simulink model "finger_model_based_control_v2"  (Simulink 6.6)
settings: Solver=ode3  StartTime=0.0  StopTime=5  FixedStep=0.01  RelTol=1e-3
undefined symbols (not defined in the file or in its folder): get
libraries: simulink x5, dspinverses x1, dspsnks4 x1
settings Model: Creator=Jadav Das  LastModifiedBy=Jadav Das
settings OptimizationCC: InlineInvariantSignals=on
settings DebuggingCC: SignalResolutionControl=TryResolveAllWithWarning  MultiTaskDSMMsg=warning  MultiTaskCondExecSysMsg=none  StrictBusMsg=None
settings RTWCC: IncludeERTFirstTime=on

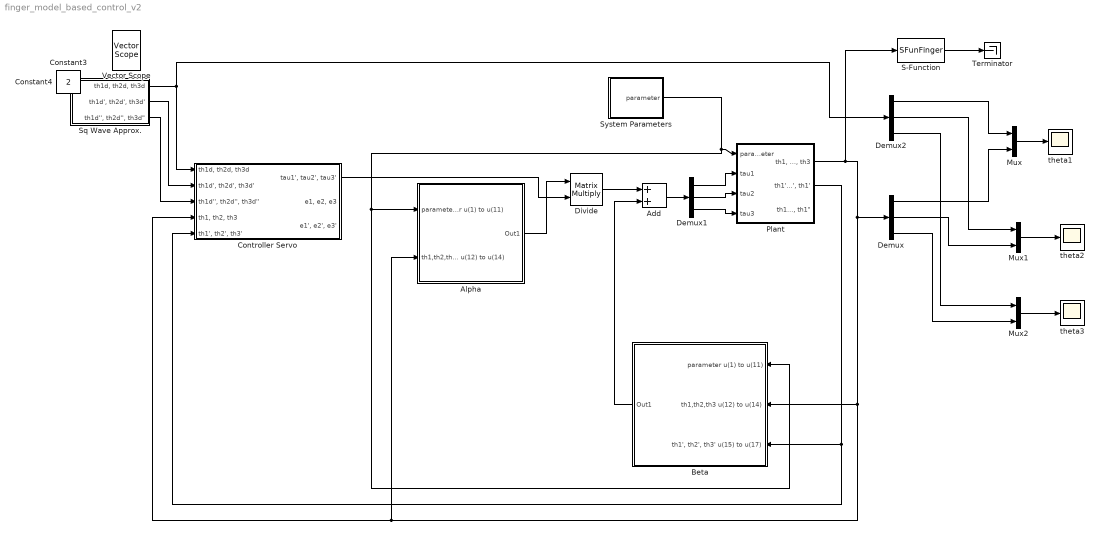
== system finger_model_based_control_v2 ==
  Add : Sum  OutScaling=2^-10
  Alpha : Subsystem
  Beta : Subsystem  Orientation=left
  Controller Servo : Subsystem
  Demux : Demux  Outputs=3
  Demux1 : Demux  Outputs=3
  Demux2 : Demux  Outputs=3
  Divide : Product  Inputs=**  Multiplication=Matrix(*)  OutScaling=2^-10
  Mux : Mux  Inputs=2
  Mux1 : Mux  Inputs=2
  Mux2 : Mux  Inputs=2
  Plant : Subsystem
  S-Function : S-Function  FunctionName=SFunFinger
  Sq Wave Approx. : Subsystem
  System Parameters : Subsystem
  Terminator : Terminator
  theta1 : Scope
      settings: TimeRange=40
  theta2 : Scope
      settings: TimeRange=40  SaveName=ScopeData2
  theta3 : Scope
      settings: TimeRange=40  SaveName=ScopeData3
  Constant3 : Constant  IOType=siggen  Value=0.5
  Constant4 : Constant  IOType=siggen  Value=2
  Vector Scope : dspsnks4/Vector Scope  IOType=viewer  DialogController=dspdialog.VectorScope  DialogControllerArgs=DataTag0  ScopeProperties=on  Domain=Time  HorizSpan=1  DisplayProperties=off  AxisGrid=off  Memory=off  FrameNumber=off  AxisLegend=off  AxisZoom=off  OpenScopeAtSimStart=on  OpenScopeImmediately=off  FigPos=get(0,'defaultfigureposition')  AxisProperties=off  XUnits=Hertz  XRange=[0...Fs/2]  InheritXIncr=on  XIncr=1  XLabel=Time  XLimit=Auto  XMin=0  XMax=1  XStart=0  YUnits=dB  YLabel=Amplitude  LineProperties=off
      settings: YMin=-10  YMax=10
  wires:
  Plant/1("th1, th2, th3") -> Demux/1, Controller Servo/4("th1, th2, th3"), Alpha/2(th1,th2,th3 u(12) to u(14)), Beta/2(th1,th2,th3 u(12) to u(14)), S-Function/1
  Demux1/1 -> Plant/2(tau1)
  Demux1/2 -> Plant/3(tau2)
  Demux1/3 -> Plant/4(tau3)
  Divide/1 -> Add/1
  Add/1 -> Demux1/1
  Plant/2("th1', th2', th1'") -> Controller Servo/5("th1', th2', th3'"), Beta/3("th1', th2', th3' u(15) to u(17)")
  Controller Servo/1("tau1', tau2', tau3'") -> Divide/2
  Sq Wave Approx./1("th1d, th2d, th3d") -> Controller Servo/1("th1d, th2d, th3d"), Demux2/1
  Sq Wave Approx./2("th1d', th2d', th3d'") -> Controller Servo/2("th1d', th2d', th3d'")
  Sq Wave Approx./3("th1d'', th2d'', th3d\"") -> Controller Servo/3("th1d'', th2d'', th3d''")
  Beta/1(Out1) -> Add/2
  Alpha/1(Out1) -> Divide/1
  Demux/1 -> Mux/2
  Mux/1 -> theta1/1
  Demux2/1 -> Mux/1
  Demux2/2 -> Mux1/1
  Demux/2 -> Mux1/2
  Mux1/1 -> theta2/1
  Demux2/3 -> Mux2/1
  Demux/3 -> Mux2/2
  Mux2/1 -> theta3/1
  S-Function/1 -> Terminator/1
  System Parameters/1(parameter) -> Beta/1(parameter u(1) to u(11)), Alpha/1(parameter u(1) to u(11)), Plant/1(parameter)

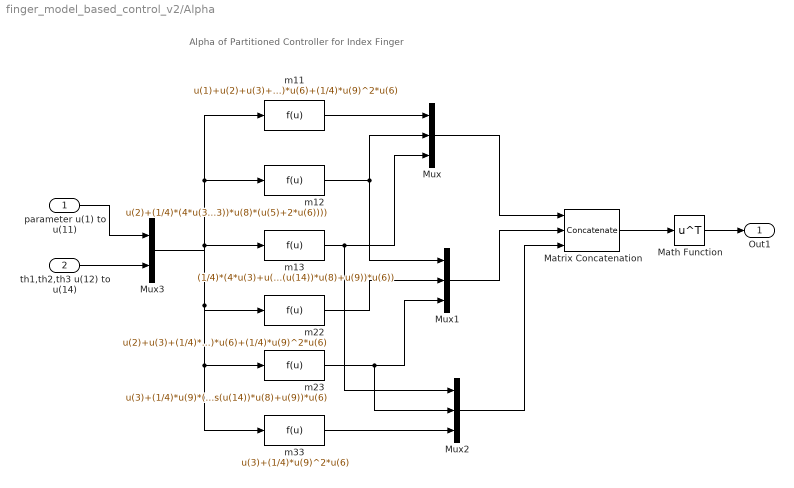
== system finger_model_based_control_v2/Alpha ==
  note: Alpha of Partitioned Controller for Index Finger
  parameter u(1) to u(11) : Inport
  th1,th2,th3 u(12) to u(14) : Inport  Port=2
  Math Function : Math  Operator=transpose  SaturateOnIntegerOverflow=on
  Matrix Concatenation : Concatenate  NumInputs=3  Mode=Multidimensional array  ConcatenateDimension=2
  Mux : Mux  Inputs=3
  Mux1 : Mux  Inputs=3
  Mux2 : Mux  Inputs=3
  Mux3 : Mux  Inputs=2
  m11 : Fcn  Expr=u(1)+u(2)+u(3)+(1/4)*u(7)^2*u(4)+u(7)^2*u(5)+cos(u(13))*u(7)*u(8)*u(5)+(1/4)*u(8)^2*u(5)+u(7)^2*u(6)+2*cos(u(13))*u(7)*u(8)*u(6)+u(8)^2*u(6)+cos(u(13)+u(14))*u(7)*u(9)*u(6)+cos(u(14))*u(8)*u(9)*u(6)+(1/4)*u(9)^2*u(6)
  m12 : Fcn  Expr=u(2)+(1/4)*(4*u(3)+u(8)^2*u(5)+4*u(8)^2*u(6)+4*cos(u(14))*u(8)*u(9)*u(6)+u(9)^2*u(6)+2*u(7)*(cos(u(13)+u(14))*u(9)*u(6)+cos(u(13))*u(8)*(u(5)+2*u(6))))
  m13 : Fcn  Expr=(1/4)*(4*u(3)+u(9)*(2*cos(u(13)+u(14))*u(7)+2*cos(u(14))*u(8)+u(9))*u(6))
  m22 : Fcn  Expr=u(2)+u(3)+(1/4)*u(8)^2*u(5)+u(8)^2*u(6)+cos(u(14))*u(8)*u(9)*u(6)+(1/4)*u(9)^2*u(6)
  m23 : Fcn  Expr=u(3)+(1/4)*u(9)*(2*cos(u(14))*u(8)+u(9))*u(6)
  m33 : Fcn  Expr=u(3)+(1/4)*u(9)^2*u(6)
  Out1 : Outport
  wires:
  m11/1 -> Mux/1
  m12/1 -> Mux1/1, Mux/2
  m13/1 -> Mux2/1, Mux/3
  Mux/1 -> Matrix Concatenation/1
  m22/1 -> Mux1/2
  m23/1 -> Mux1/3, Mux2/2
  Mux1/1 -> Matrix Concatenation/2
  m33/1 -> Mux2/3
  Mux2/1 -> Matrix Concatenation/3
  Matrix Concatenation/1 -> Math Function/1
  Math Function/1 -> Out1/1
  parameter u(1) to u(11)/1 -> Mux3/1
  th1,th2,th3 u(12) to u(14)/1 -> Mux3/2
  Mux3/1 -> m11/1, m12/1, m13/1, m22/1, m23/1, m33/1

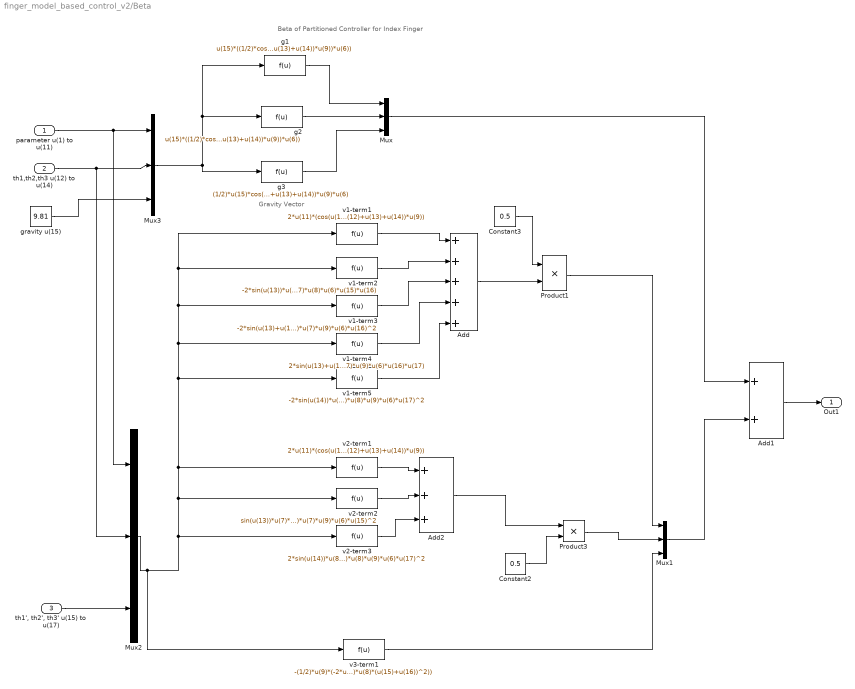
== system finger_model_based_control_v2/Beta ==
  note: Beta of Partitioned Controller for Index Finger
  note: Gravity Vector
  parameter u(1) to u(11) : Inport
  th1,th2,th3 u(12) to u(14) : Inport  Port=2
  "th1', th2', th3' u(15) to u(17)" : Inport  Port=3
  Add : Sum  Inputs=+++++  OutScaling=2^-10
  Add1 : Sum  OutScaling=2^-10
  Add2 : Sum  Inputs=+++  OutScaling=2^-10
  Constant2 : Constant  Value=0.5
  Constant3 : Constant  Value=0.5
  Mux{,1..3} (4 alike) : Mux  Inputs=3
  Product1 : Product  RndMeth=Zero
  Product3 : Product  RndMeth=Zero
  g1 : Fcn  Expr=u(15)*((1/2)*cos(u(12))*u(7)*u(4)+(cos(u(12))*u(7)+(1/2)*cos(u(12)+u(13))*u(8))*u(5)+(cos(u(12))*u(7)+cos(u(12)+u(13))*u(8)+(1/2)*cos(u(12)+u(13)+u(14))*u(9))*u(6))
  g2 : Fcn  Expr=u(15)*((1/2)*cos(u(12)+u(13))*u(8)*u(5)+(cos(u(12)+u(13))*u(8)+(1/2)*cos(u(12)+u(13)+u(14))*u(9))*u(6))
  g3 : Fcn  Expr=(1/2)*u(15)*cos(u(12)+u(13)+u(14))*u(9)*u(6)
  gravity u(15) : Constant  Value=9.81
  v1-term1 : Fcn  Expr=2*u(11)*(cos(u(12))*u(7)+cos(u(12)+u(13))*u(8)+cos(u(12)+u(13)+u(14))*u(9))-2*u(10)*(sin(u(12))*u(7)+sin(u(12)+u(13))*u(8)+sin(u(12)+u(13)+u(14))*u(9))
  v1-term2 : Fcn  Expr=-2*sin(u(13))*u(7)*u(8)*u(6)*u(15)^2-2*sin(u(14))*u(7)*u(8)*u(6)*u(15)^2-2*sin(u(13))*u(7)*u(8)*u(5)*u(15)*u(16)-4*sin(u(13))*u(7)*u(8)*u(6)*u(15)*u(16)
  v1-term3 : Fcn  Expr=-2*sin(u(13)+u(14))*u(7)*u(9)*u(6)*u(15)*u(16)-sin(u(13))*u(7)*u(8)*u(5)*u(16)^2-2*sin(u(13))*u(7)*u(8)*u(6)*u(16)^2-sin(u(13)+u(14))*u(7)*u(9)*u(6)*u(16)^2
  v1-term4 : Fcn  Expr=2*sin(u(13)+u(14))*u(7)*u(9)*u(6)*u(15)*u(17)-2*sin(u(14))*u(8)*u(9)*u(6)*u(15)*u(17)-2*sin(u(13)+u(14))*u(7)*u(9)*u(6)*u(16)*u(17)
  v1-term5 : Fcn  Expr=-2*sin(u(14))*u(8)*u(9)*u(6)*u(16)*u(17)-sin(u(13)+u(14))*u(7)*u(9)*u(6)*u(17)^2-sin(u(14))*u(8)*u(9)*u(6)*u(17)^2
  v2-term1 : Fcn  Expr=2*u(11)*(cos(u(12)+u(13))*u(8)+cos(u(12)+u(13)+u(14))*u(9))-2*u(10)*(sin(u(12)+u(13))*u(8)+sin(u(12)+u(13)+u(14))*u(9))
  v2-term2 : Fcn  Expr=sin(u(13))*u(7)*u(8)*u(5)*u(15)^2+2*sin(u(13))*u(7)*u(8)*u(6)*u(15)^2+sin(u(13)+u(14))*u(7)*u(9)*u(6)*u(15)^2
  v2-term3 : Fcn  Expr=2*sin(u(14))*u(8)*u(9)*u(6)*u(15)*u(17)-2*sin(u(14))*u(8)*u(9)*u(6)*u(16)*u(17)-sin(u(14))*u(8)*u(9)*u(6)*u(17)^2
  v3-term1 : Fcn  Expr=-(1/2)*u(9)*(-2*u(11)*cos(u(12)+u(13)+u(14))+2*u(10)*sin(u(12)+u(13)+u(14))-u(6)*(sin(u(13)+u(14))*u(7)*u(15)^2+sin(u(14))*u(8)*(u(15)+u(16))^2))
  Out1 : Outport
  wires:
  g1/1 -> Mux/1
  g2/1 -> Mux/2
  g3/1 -> Mux/3
  parameter u(1) to u(11)/1 -> Mux3/1, Mux2/1
  th1,th2,th3 u(12) to u(14)/1 -> Mux3/2, Mux2/2
  Mux3/1 -> g3/1, g2/1, g1/1
  gravity u(15)/1 -> Mux3/3
  Mux2/1 -> v2-term1/1, v1-term1/1, v1-term2/1, v1-term3/1, v1-term4/1, v1-term5/1, v2-term2/1, v2-term3/1, v3-term1/1
  v1-term1/1 -> Add/1
  v2-term1/1 -> Add2/1
  v2-term2/1 -> Add2/2
  Product3/1 -> Mux1/2
  Constant2/1 -> Product3/2
  "th1', th2', th3' u(15) to u(17)"/1 -> Mux2/3
  v1-term2/1 -> Add/2
  v1-term3/1 -> Add/3
  v1-term4/1 -> Add/4
  v1-term5/1 -> Add/5
  Add/1 -> Product1/2
  Constant3/1 -> Product1/1
  Product1/1 -> Mux1/1
  v2-term3/1 -> Add2/3
  Add2/1 -> Product3/1
  v3-term1/1 -> Mux1/3
  Mux1/1 -> Add1/2
  Mux/1 -> Add1/1
  Add1/1 -> Out1/1

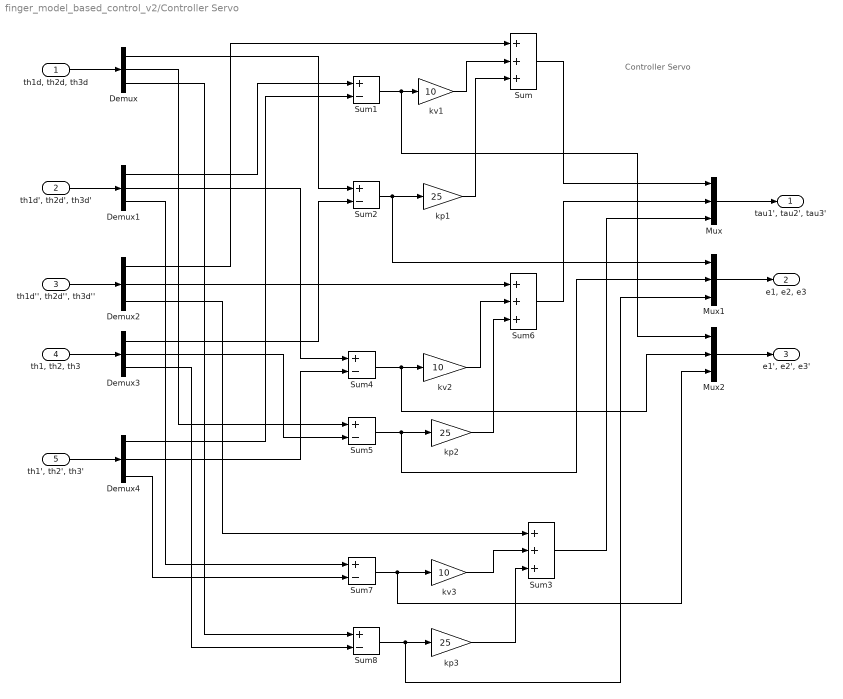
== system finger_model_based_control_v2/Controller Servo ==
  note: Controller Servo
  "th1d, th2d, th3d" : Inport
  "th1d', th2d', th3d'" : Inport  Port=2
  "th1d'', th2d'', th3d''" : Inport  Port=3
  "th1, th2, th3" : Inport  Port=4
  "th1', th2', th3'" : Inport  Port=5
  Demux{,1..4} (5 alike) : Demux  Outputs=3
  Mux : Mux  Inputs=3
  Mux1 : Mux  Inputs=3
  Mux2 : Mux  Inputs=3
  Sum : Sum  Inputs=+++  SaturateOnIntegerOverflow=on  InputSameDT=on
  Sum{1..2,4..5,7..8} (6 alike) : Sum  Inputs=+-  SaturateOnIntegerOverflow=on  InputSameDT=on
  Sum3 : Sum  Inputs=+++  SaturateOnIntegerOverflow=on  InputSameDT=on
  Sum6 : Sum  Inputs=+++  SaturateOnIntegerOverflow=on  InputSameDT=on
  kp1 : Gain  Gain=25  SaturateOnIntegerOverflow=on
  kp2 : Gain  Gain=25  SaturateOnIntegerOverflow=on
  kp3 : Gain  Gain=25  SaturateOnIntegerOverflow=on
  kv1 : Gain  Gain=10  SaturateOnIntegerOverflow=on
  kv2 : Gain  Gain=10  SaturateOnIntegerOverflow=on
  kv3 : Gain  Gain=10  SaturateOnIntegerOverflow=on
  "tau1', tau2', tau3'" : Outport
  "e1, e2, e3" : Outport  Port=2
  "e1', e2', e3'" : Outport  Port=3
  wires:
  Sum2/1 -> kp1/1, Mux1/1
  kp1/1 -> Sum/3
  Sum1/1 -> kv1/1, Mux2/1
  kv1/1 -> Sum/2
  Sum4/1 -> kv2/1, Mux2/2
  kv2/1 -> Sum6/2
  Sum5/1 -> kp2/1, Mux1/2
  kp2/1 -> Sum6/3
  Sum/1 -> Mux/1
  Sum6/1 -> Mux/2
  Mux/1 -> "tau1', tau2', tau3'"/1
  "th1d, th2d, th3d"/1 -> Demux/1
  "th1d', th2d', th3d'"/1 -> Demux1/1
  "th1d'', th2d'', th3d''"/1 -> Demux2/1
  "th1, th2, th3"/1 -> Demux3/1
  "th1', th2', th3'"/1 -> Demux4/1
  Demux2/1 -> Sum/1
  Demux1/1 -> Sum1/1
  Demux4/1 -> Sum1/2
  Demux/1 -> Sum2/1
  Demux2/2 -> Sum6/1
  Demux1/2 -> Sum4/1
  Demux4/2 -> Sum4/2
  Demux/2 -> Sum5/1
  Demux3/2 -> Sum5/2
  Demux3/1 -> Sum2/2
  Mux1/1 -> "e1, e2, e3"/1
  Mux2/1 -> "e1', e2', e3'"/1
  Demux4/3 -> Sum7/2
  Sum7/1 -> kv3/1, Mux2/3
  kv3/1 -> Sum3/2
  Demux/3 -> Sum8/1
  Demux3/3 -> Sum8/2
  Sum8/1 -> kp3/1, Mux1/3
  kp3/1 -> Sum3/3
  Sum3/1 -> Mux/3
  Demux1/3 -> Sum7/1
  Demux2/3 -> Sum3/1

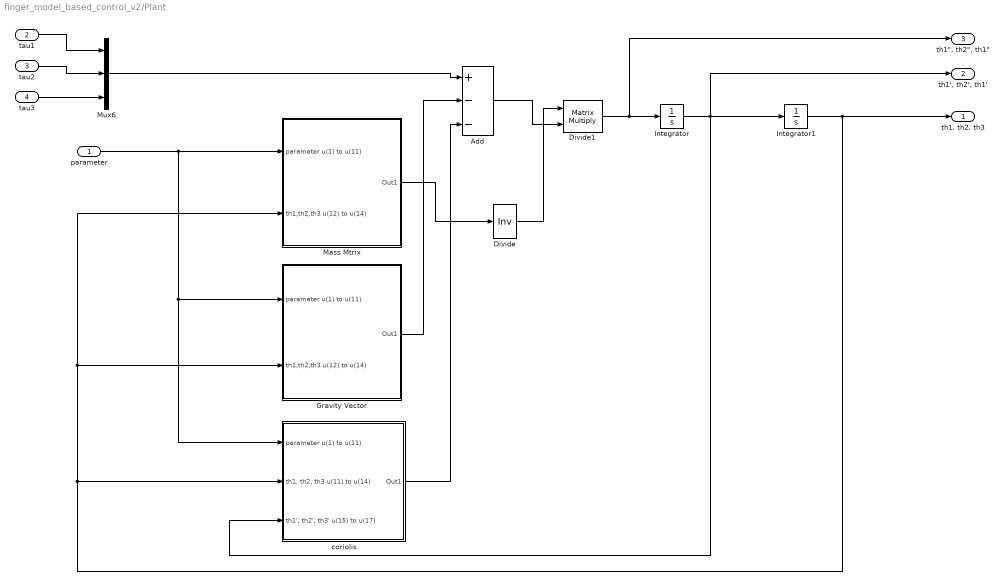
== system finger_model_based_control_v2/Plant ==
  parameter : Inport
  tau1 : Inport  Port=2
  tau2 : Inport  Port=3
  tau3 : Inport  Port=4
  Add : Sum  Inputs=+--  OutScaling=2^-10
  Divide : Product  Inputs=/  Multiplication=Matrix(*)  OutScaling=2^-10
  Divide1 : Product  Inputs=**  Multiplication=Matrix(*)  OutScaling=2^-10
  Gravity Vector : Subsystem
  Integrator : Integrator
  Integrator1 : Integrator  InitialCondition=[0.1, 0.1, 0.1]
  Mass Mtrix : Subsystem
  Mux6 : Mux  Inputs=3
  coriolis : Subsystem
  "th1, th2, th3" : Outport
  "th1', th2', th1'" : Outport  Port=2
  "th1\", th2\", th1\"" : Outport  Port=3
  wires:
  Gravity Vector/1(Out1) -> Add/2
  Mass Mtrix/1(Out1) -> Divide/1
  Divide/1 -> Divide1/1
  Add/1 -> Divide1/2
  Divide1/1 -> Integrator/1, "th1\", th2\", th1\""/1
  Integrator/1 -> Integrator1/1, "th1', th2', th1'"/1, coriolis/3("th1', th2', th3' u(15) to u(17)")
  Integrator1/1 -> "th1, th2, th3"/1, Mass Mtrix/2(th1,th2,th3 u(12) to u(14)), Gravity Vector/2(th1,th2,th3 u(12) to u(14)), coriolis/2("th1, th2, th3 u(11) to u(14)")
  Mux6/1 -> Add/1
  tau1/1 -> Mux6/1
  tau2/1 -> Mux6/2
  tau3/1 -> Mux6/3
  coriolis/1(Out1) -> Add/3
  parameter/1 -> Mass Mtrix/1(parameter u(1) to u(11)), Gravity Vector/1(parameter u(1) to u(11)), coriolis/1(parameter u(1) to u(11))

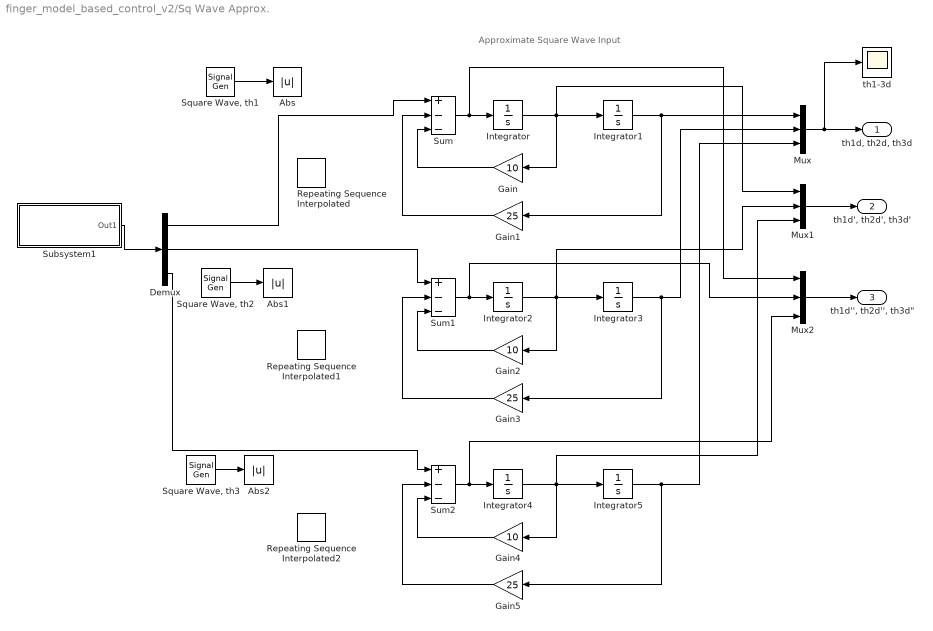
== system finger_model_based_control_v2/Sq Wave Approx. ==
  note: Approximate Square Wave Input
  Abs : Abs
  Abs1 : Abs
  Abs2 : Abs
  Demux : Demux  Outputs=3
  Gain : Gain  Orientation=left  Gain=10  SaturateOnIntegerOverflow=on
  Gain1 : Gain  Orientation=left  Gain=25  SaturateOnIntegerOverflow=on
  Gain2 : Gain  Orientation=left  Gain=10  SaturateOnIntegerOverflow=on
  Gain3 : Gain  Orientation=left  Gain=25  SaturateOnIntegerOverflow=on
  Gain4 : Gain  Orientation=left  Gain=10  SaturateOnIntegerOverflow=on
  Gain5 : Gain  Orientation=left  Gain=25  SaturateOnIntegerOverflow=on
  Integrator{,1..5} (6 alike) : Integrator
  Mux : Mux  Inputs=3
  Mux1 : Mux  Inputs=3
  Mux2 : Mux  Inputs=3
  Repeating Sequence Interpolated : simulink/Sources/Repeating Sequence Interpolated  SystemSampleTime=-1  OutValues=[0 90*pi/180 0 0].'  TimeValues=[0 1 2 3].'  LookUpMeth=Interpolation-Use End Values  tsamp=0.01  OutputDataTypeScalingMode=Specify via dialog  OutDataType=float('double')  OutScaling=2^-10
  Repeating Sequence Interpolated1 : simulink/Sources/Repeating Sequence Interpolated  SystemSampleTime=-1  OutValues=[0*pi/180 190*pi/180 45*pi/180 0*pi/180].'  TimeValues=[0 1 2 3].'  LookUpMeth=Interpolation-Use End Values  tsamp=0.01  OutputDataTypeScalingMode=Specify via dialog  OutDataType=float('double')  OutScaling=2^-10
  Repeating Sequence Interpolated2 : simulink/Sources/Repeating Sequence Interpolated  SystemSampleTime=-1  OutValues=[pi 90*pi/180 pi pi].'  TimeValues=[0 1 2 3].'  LookUpMeth=Interpolation-Use End Values  tsamp=0.01  OutputDataTypeScalingMode=Specify via dialog  OutDataType=float('double')  OutScaling=2^-10
  "Square Wave, th1" : SignalGenerator  Amplitude=10  Frequency=.2
  "Square Wave, th2" : SignalGenerator  Amplitude=10  Frequency=.2
  "Square Wave, th3" : SignalGenerator  Amplitude=10  Frequency=.2
  Subsystem1 : Subsystem
  Sum : Sum  Inputs=+--  SaturateOnIntegerOverflow=on  InputSameDT=on
  Sum1 : Sum  Inputs=+--  SaturateOnIntegerOverflow=on  InputSameDT=on
  Sum2 : Sum  Inputs=+--  SaturateOnIntegerOverflow=on  InputSameDT=on
  th1-3d : Scope
  "th1d, th2d, th3d" : Outport
  "th1d', th2d', th3d'" : Outport  Port=2
  "th1d'', th2d'', th3d\"" : Outport  Port=3
  wires:
  Mux2/1 -> "th1d'', th2d'', th3d\""/1
  Mux1/1 -> "th1d', th2d', th3d'"/1
  Mux/1 -> "th1d, th2d, th3d"/1, th1-3d/1
  Sum1/1 -> Mux2/2, Integrator2/1
  Integrator3/1 -> Mux/2, Gain3/1
  Gain3/1 -> Sum1/2
  Gain2/1 -> Sum1/3
  Integrator2/1 -> Mux1/2, Gain2/1, Integrator3/1
  Sum/1 -> Mux2/1, Integrator/1
  Integrator1/1 -> Mux/1, Gain1/1
  Gain1/1 -> Sum/2
  Gain/1 -> Sum/3
  Integrator/1 -> Mux1/1, Gain/1, Integrator1/1
  Sum2/1 -> Integrator4/1, Mux2/3
  Integrator5/1 -> Gain5/1, Mux/3
  Gain5/1 -> Sum2/2
  Gain4/1 -> Sum2/3
  Integrator4/1 -> Integrator5/1, Gain4/1, Mux1/3
  "Square Wave, th1"/1 -> Abs/1
  "Square Wave, th2"/1 -> Abs1/1
  "Square Wave, th3"/1 -> Abs2/1
  Subsystem1/1(Out1) -> Demux/1
  Demux/1 -> Sum/1
  Demux/2 -> Sum1/1
  Demux/3 -> Sum2/1

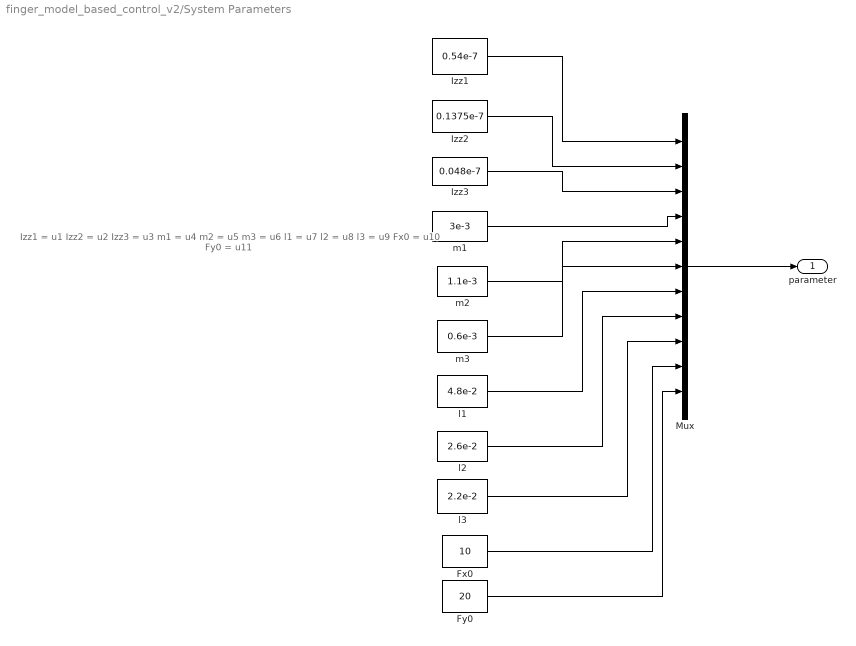
== system finger_model_based_control_v2/System Parameters ==
  note: Izz1 = u1
      | Izz2 = u2
      | Izz3 = u3
      | m1 = u4
      | m2 = u5
      | m3 = u6
      | l1 = u7
      | l2 = u8
      | l3 = u9
      | Fx0 = u10
      | Fy0 = u11
  Fx0 : Constant  Value=10
  Fy0 : Constant  Value=20
  Izz1 : Constant  Value=0.54e-7
  Izz2 : Constant  Value=0.1375e-7
  Izz3 : Constant  Value=0.048e-7
  Mux : Mux  Inputs=11
  l1 : Constant  Value=4.8e-2
  l2 : Constant  Value=2.6e-2
  l3 : Constant  Value=2.2e-2
  m1 : Constant  Value=3e-3
  m2 : Constant  Value=1.1e-3
  m3 : Constant  Value=0.6e-3
  parameter : Outport
  wires:
  Mux/1 -> parameter/1
  Izz1/1 -> Mux/1
  Izz2/1 -> Mux/2
  Izz3/1 -> Mux/3
  m1/1 -> Mux/4
  m2/1 -> Mux/5
  m3/1 -> Mux/6
  l1/1 -> Mux/7
  l2/1 -> Mux/8
  l3/1 -> Mux/9
  Fx0/1 -> Mux/10
  Fy0/1 -> Mux/11

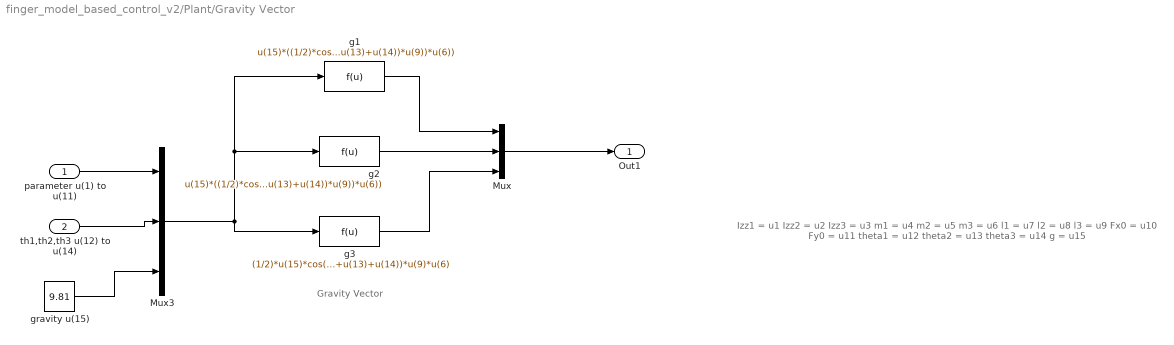
== system finger_model_based_control_v2/Plant/Gravity Vector ==
  note: Gravity Vector
  note: Izz1 = u1
      | Izz2 = u2
      | Izz3 = u3
      | m1 = u4
      | m2 = u5
      | m3 = u6
      | l1 = u7
      | l2 = u8
      | l3 = u9
      | Fx0 = u10
      | Fy0 = u11
      | theta1 = u12
      | theta2 = u13
      | theta3 = u14
      | g = u15
  parameter u(1) to u(11) : Inport
  th1,th2,th3 u(12) to u(14) : Inport  Port=2
  Mux : Mux  Inputs=3
  Mux3 : Mux  Inputs=3
  g1 : Fcn  Expr=u(15)*((1/2)*cos(u(12))*u(7)*u(4)+(cos(u(12))*u(7)+(1/2)*cos(u(12)+u(13))*u(8))*u(5)+(cos(u(12))*u(7)+cos(u(12)+u(13))*u(8)+(1/2)*cos(u(12)+u(13)+u(14))*u(9))*u(6))
  g2 : Fcn  Expr=u(15)*((1/2)*cos(u(12)+u(13))*u(8)*u(5)+(cos(u(12)+u(13))*u(8)+(1/2)*cos(u(12)+u(13)+u(14))*u(9))*u(6))
  g3 : Fcn  Expr=(1/2)*u(15)*cos(u(12)+u(13)+u(14))*u(9)*u(6)
  gravity u(15) : Constant  Value=9.81
  Out1 : Outport
  wires:
  g1/1 -> Mux/1
  g2/1 -> Mux/2
  g3/1 -> Mux/3
  Mux/1 -> Out1/1
  parameter u(1) to u(11)/1 -> Mux3/1
  th1,th2,th3 u(12) to u(14)/1 -> Mux3/2
  Mux3/1 -> g3/1, g2/1, g1/1
  gravity u(15)/1 -> Mux3/3

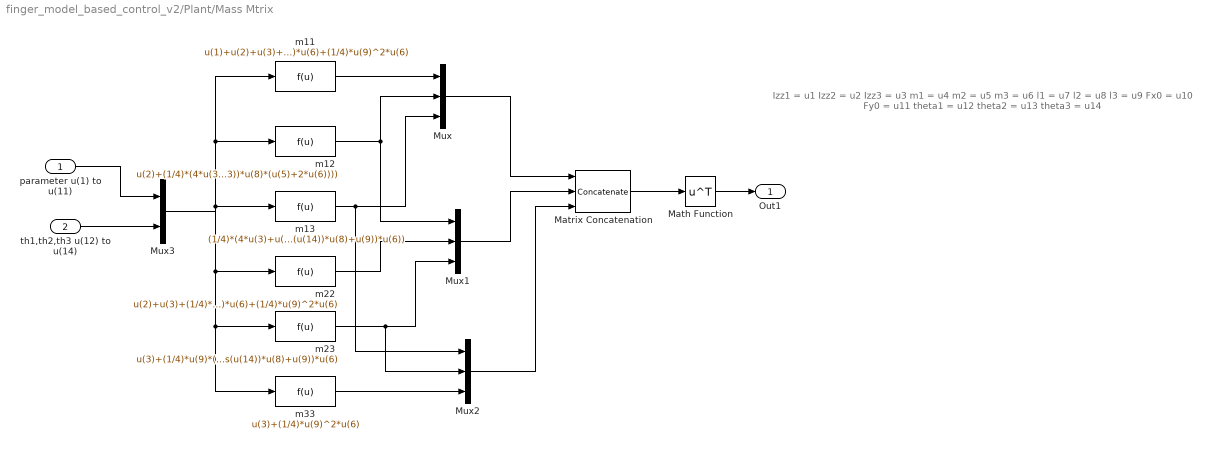
== system finger_model_based_control_v2/Plant/Mass Mtrix ==
  note: Izz1 = u1
      | Izz2 = u2
      | Izz3 = u3
      | m1 = u4
      | m2 = u5
      | m3 = u6
      | l1 = u7
      | l2 = u8
      | l3 = u9
      | Fx0 = u10
      | Fy0 = u11
      | theta1 = u12
      | theta2 = u13
      | theta3 = u14
  parameter u(1) to u(11) : Inport
  th1,th2,th3 u(12) to u(14) : Inport  Port=2
  Math Function : Math  Operator=transpose  SaturateOnIntegerOverflow=on
  Matrix Concatenation : Concatenate  NumInputs=3  Mode=Multidimensional array  ConcatenateDimension=2
  Mux : Mux  Inputs=3
  Mux1 : Mux  Inputs=3
  Mux2 : Mux  Inputs=3
  Mux3 : Mux  Inputs=2
  m11 : Fcn  Expr=u(1)+u(2)+u(3)+(1/4)*u(7)^2*u(4)+u(7)^2*u(5)+cos(u(13))*u(7)*u(8)*u(5)+(1/4)*u(8)^2*u(5)+u(7)^2*u(6)+2*cos(u(13))*u(7)*u(8)*u(6)+u(8)^2*u(6)+cos(u(13)+u(14))*u(7)*u(9)*u(6)+cos(u(14))*u(8)*u(9)*u(6)+(1/4)*u(9)^2*u(6)
  m12 : Fcn  Expr=u(2)+(1/4)*(4*u(3)+u(8)^2*u(5)+4*u(8)^2*u(6)+4*cos(u(14))*u(8)*u(9)*u(6)+u(9)^2*u(6)+2*u(7)*(cos(u(13)+u(14))*u(9)*u(6)+cos(u(13))*u(8)*(u(5)+2*u(6))))
  m13 : Fcn  Expr=(1/4)*(4*u(3)+u(9)*(2*cos(u(13)+u(14))*u(7)+2*cos(u(14))*u(8)+u(9))*u(6))
  m22 : Fcn  Expr=u(2)+u(3)+(1/4)*u(8)^2*u(5)+u(8)^2*u(6)+cos(u(14))*u(8)*u(9)*u(6)+(1/4)*u(9)^2*u(6)
  m23 : Fcn  Expr=u(3)+(1/4)*u(9)*(2*cos(u(14))*u(8)+u(9))*u(6)
  m33 : Fcn  Expr=u(3)+(1/4)*u(9)^2*u(6)
  Out1 : Outport
  wires:
  m11/1 -> Mux/1
  m12/1 -> Mux1/1, Mux/2
  m13/1 -> Mux2/1, Mux/3
  Mux/1 -> Matrix Concatenation/1
  m22/1 -> Mux1/2
  m23/1 -> Mux1/3, Mux2/2
  Mux1/1 -> Matrix Concatenation/2
  m33/1 -> Mux2/3
  Mux2/1 -> Matrix Concatenation/3
  Matrix Concatenation/1 -> Math Function/1
  Math Function/1 -> Out1/1
  parameter u(1) to u(11)/1 -> Mux3/1
  th1,th2,th3 u(12) to u(14)/1 -> Mux3/2
  Mux3/1 -> m11/1, m12/1, m13/1, m22/1, m23/1, m33/1

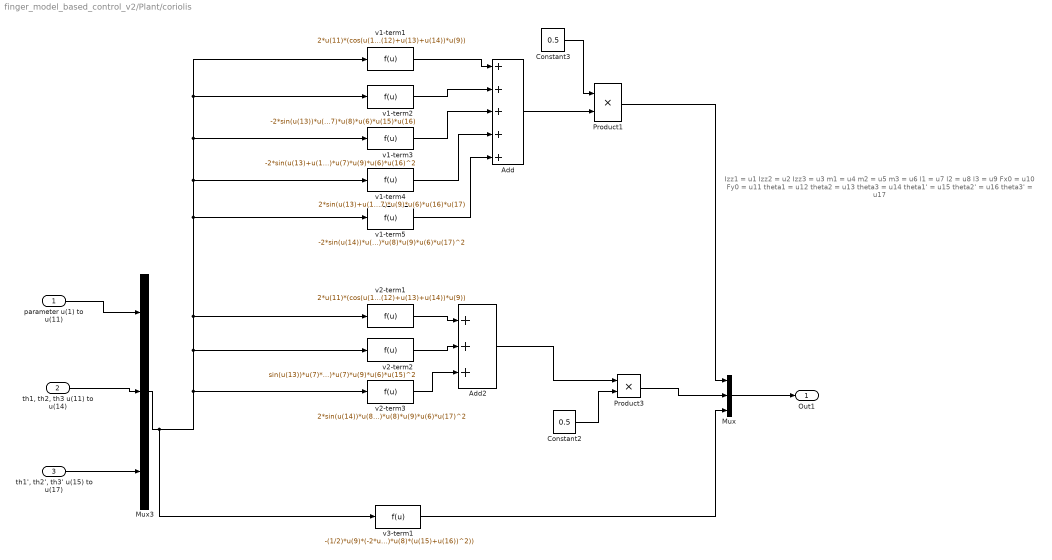
== system finger_model_based_control_v2/Plant/coriolis ==
  note: Izz1 = u1
      | Izz2 = u2
      | Izz3 = u3
      | m1 = u4
      | m2 = u5
      | m3 = u6
      | l1 = u7
      | l2 = u8
      | l3 = u9
      | Fx0 = u10
      | Fy0 = u11
      | theta1 = u12
      | theta2 = u13
      | theta3 = u14
      | theta1' = u15
      | theta2' = u16
      | theta3' = u17
  parameter u(1) to u(11) : Inport
  "th1, th2, th3 u(11) to u(14)" : Inport  Port=2
  "th1', th2', th3' u(15) to u(17)" : Inport  Port=3
  Add : Sum  Inputs=+++++  OutScaling=2^-10
  Add2 : Sum  Inputs=+++  OutScaling=2^-10
  Constant2 : Constant  Value=0.5
  Constant3 : Constant  Value=0.5
  Mux : Mux  Inputs=3
  Mux3 : Mux  Inputs=3
  Product1 : Product  RndMeth=Zero
  Product3 : Product  RndMeth=Zero
  v1-term1 : Fcn  Expr=2*u(11)*(cos(u(12))*u(7)+cos(u(12)+u(13))*u(8)+cos(u(12)+u(13)+u(14))*u(9))-2*u(10)*(sin(u(12))*u(7)+sin(u(12)+u(13))*u(8)+sin(u(12)+u(13)+u(14))*u(9))
  v1-term2 : Fcn  Expr=-2*sin(u(13))*u(7)*u(8)*u(6)*u(15)^2-2*sin(u(14))*u(7)*u(8)*u(6)*u(15)^2-2*sin(u(13))*u(7)*u(8)*u(5)*u(15)*u(16)-4*sin(u(13))*u(7)*u(8)*u(6)*u(15)*u(16)
  v1-term3 : Fcn  Expr=-2*sin(u(13)+u(14))*u(7)*u(9)*u(6)*u(15)*u(16)-sin(u(13))*u(7)*u(8)*u(5)*u(16)^2-2*sin(u(13))*u(7)*u(8)*u(6)*u(16)^2-sin(u(13)+u(14))*u(7)*u(9)*u(6)*u(16)^2
  v1-term4 : Fcn  Expr=2*sin(u(13)+u(14))*u(7)*u(9)*u(6)*u(15)*u(17)-2*sin(u(14))*u(8)*u(9)*u(6)*u(15)*u(17)-2*sin(u(13)+u(14))*u(7)*u(9)*u(6)*u(16)*u(17)
  v1-term5 : Fcn  Expr=-2*sin(u(14))*u(8)*u(9)*u(6)*u(16)*u(17)-sin(u(13)+u(14))*u(7)*u(9)*u(6)*u(17)^2-sin(u(14))*u(8)*u(9)*u(6)*u(17)^2
  v2-term1 : Fcn  Expr=2*u(11)*(cos(u(12)+u(13))*u(8)+cos(u(12)+u(13)+u(14))*u(9))-2*u(10)*(sin(u(12)+u(13))*u(8)+sin(u(12)+u(13)+u(14))*u(9))
  v2-term2 : Fcn  Expr=sin(u(13))*u(7)*u(8)*u(5)*u(15)^2+2*sin(u(13))*u(7)*u(8)*u(6)*u(15)^2+sin(u(13)+u(14))*u(7)*u(9)*u(6)*u(15)^2
  v2-term3 : Fcn  Expr=2*sin(u(14))*u(8)*u(9)*u(6)*u(15)*u(17)-2*sin(u(14))*u(8)*u(9)*u(6)*u(16)*u(17)-sin(u(14))*u(8)*u(9)*u(6)*u(17)^2
  v3-term1 : Fcn  Expr=-(1/2)*u(9)*(-2*u(11)*cos(u(12)+u(13)+u(14))+2*u(10)*sin(u(12)+u(13)+u(14))-u(6)*(sin(u(13)+u(14))*u(7)*u(15)^2+sin(u(14))*u(8)*(u(15)+u(16))^2))
  Out1 : Outport
  wires:
  Mux3/1 -> v2-term1/1, v1-term1/1, v1-term2/1, v1-term3/1, v1-term4/1, v1-term5/1, v2-term2/1, v2-term3/1, v3-term1/1
  "th1, th2, th3 u(11) to u(14)"/1 -> Mux3/2
  parameter u(1) to u(11)/1 -> Mux3/1
  v1-term1/1 -> Add/1
  v2-term1/1 -> Add2/1
  v2-term2/1 -> Add2/2
  Product3/1 -> Mux/2
  Mux/1 -> Out1/1
  Constant2/1 -> Product3/2
  "th1', th2', th3' u(15) to u(17)"/1 -> Mux3/3
  v1-term2/1 -> Add/2
  v1-term3/1 -> Add/3
  v1-term4/1 -> Add/4
  v1-term5/1 -> Add/5
  Add/1 -> Product1/2
  Constant3/1 -> Product1/1
  Product1/1 -> Mux/1
  v2-term3/1 -> Add2/3
  Add2/1 -> Product3/1
  v3-term1/1 -> Mux/3

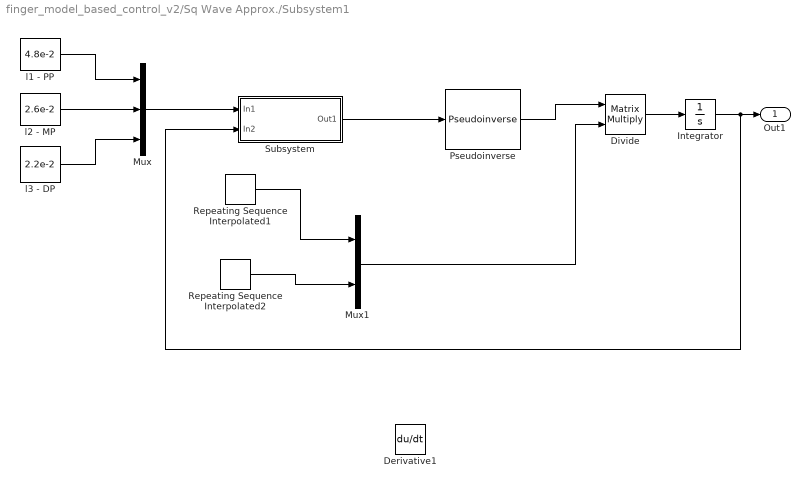
== system finger_model_based_control_v2/Sq Wave Approx./Subsystem1 ==
  Derivative1 : Derivative
  Divide : Product  Inputs=**  Multiplication=Matrix(*)  OutScaling=2^-10
  Integrator : Integrator
  Mux : Mux  Inputs=3
  Mux1 : Mux  Inputs=2
  Pseudoinverse : dspinverses/Pseudoinverse  wanterr=off
  Repeating Sequence Interpolated1 : simulink/Sources/Repeating Sequence Interpolated  SystemSampleTime=-1  OutValues=[0.08 0.06 0.04 0.06 0.08].'  TimeValues=[0 1 2 3 4].'  LookUpMeth=Interpolation-Use End Values  tsamp=0.01  OutputDataTypeScalingMode=Specify via dialog  OutDataType=float('double')  OutScaling=2^-10
  Repeating Sequence Interpolated2 : simulink/Sources/Repeating Sequence Interpolated  SystemSampleTime=-1  OutValues=[0.05 0.05 0.05 0.05 0.05].'  TimeValues=[0 1 2 3 4].'  LookUpMeth=Interpolation-Use End Values  tsamp=0.01  OutputDataTypeScalingMode=Specify via dialog  OutDataType=float('double')  OutScaling=2^-10
  Subsystem : Subsystem
  l1 - PP : Constant  Value=4.8e-2
  l2 - MP : Constant  Value=2.6e-2
  l3 - DP : Constant  Value=2.2e-2
  Out1 : Outport
  wires:
  l1 - PP/1 -> Mux/1
  l2 - MP/1 -> Mux/2
  l3 - DP/1 -> Mux/3
  Mux/1 -> Subsystem/1(In1)
  Subsystem/1(Out1) -> Pseudoinverse/1
  Pseudoinverse/1 -> Divide/1
  Mux1/1 -> Divide/2
  Divide/1 -> Integrator/1
  Integrator/1 -> Subsystem/2(In2), Out1/1
  Repeating Sequence Interpolated2/1 -> Mux1/2
  Repeating Sequence Interpolated1/1 -> Mux1/1

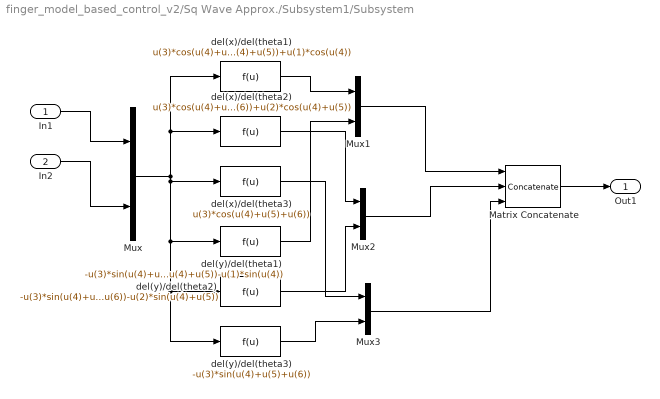
== system finger_model_based_control_v2/Sq Wave Approx./Subsystem1/Subsystem ==
  In1 : Inport
  In2 : Inport  Port=2
  Matrix Concatenate : Concatenate  NumInputs=3  Mode=Multidimensional array  ConcatenateDimension=2
  Mux{,1..3} (4 alike) : Mux  Inputs=2
  del(x)/del(theta1) : Fcn  Expr=u(3)*cos(u(4)+u(5)+u(6))+u(2)*cos(u(4)+u(5))+u(1)*cos(u(4))
  del(x)/del(theta2) : Fcn  Expr=u(3)*cos(u(4)+u(5)+u(6))+u(2)*cos(u(4)+u(5))
  del(x)/del(theta3) : Fcn  Expr=u(3)*cos(u(4)+u(5)+u(6))
  del(y)/del(theta1) : Fcn  Expr=-u(3)*sin(u(4)+u(5)+u(6))-u(2)*sin(u(4)+u(5))-u(1)*sin(u(4))
  del(y)/del(theta2) : Fcn  Expr=-u(3)*sin(u(4)+u(5)+u(6))-u(2)*sin(u(4)+u(5))
  del(y)/del(theta3) : Fcn  Expr=-u(3)*sin(u(4)+u(5)+u(6))
  Out1 : Outport
  wires:
  In1/1 -> Mux/1
  In2/1 -> Mux/2
  Mux/1 -> del(x)/del(theta1)/1, del(x)/del(theta2)/1, del(x)/del(theta3)/1, del(y)/del(theta1)/1, del(y)/del(theta2)/1, del(y)/del(theta3)/1
  Matrix Concatenate/1 -> Out1/1
  del(x)/del(theta1)/1 -> Mux1/1
  del(y)/del(theta1)/1 -> Mux1/2
  del(x)/del(theta2)/1 -> Mux2/1
  del(x)/del(theta3)/1 -> Mux3/1
  del(y)/del(theta2)/1 -> Mux2/2
  del(y)/del(theta3)/1 -> Mux3/2
  Mux1/1 -> Matrix Concatenate/1
  Mux2/1 -> Matrix Concatenate/2
  Mux3/1 -> Matrix Concatenate/3
